simulink model "BLDC_System_Level"  (R2022b)
settings: Solver=FixedStepAuto  StartTime=0.0  StopTime=10.0  RelTol=1e-3
PreLoadFcn:
  | init_params
InitFcn:
  | init_params
undefined symbols (not defined in the file): V_dc
settings Model: Creator=Ahmed Aboeita  LastModifiedBy=Ahmed Aboeita

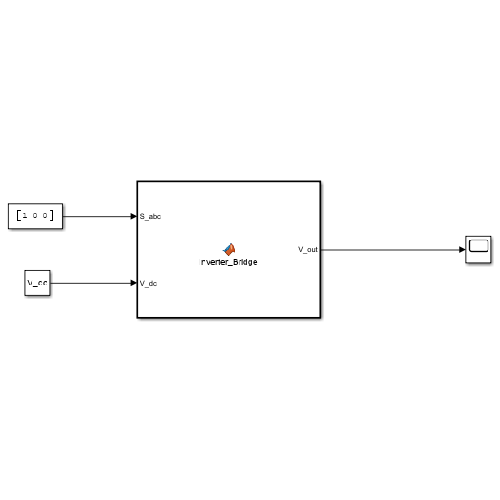
[thumbnail: Simulink's stored preview of the top-level diagram]
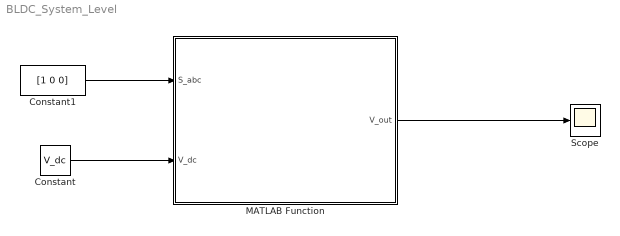
== system BLDC_System_Level ==
  Constant : Constant  Value=V_dc
  Constant1 : Constant  Value=[1 0 0]
  MATLAB Function : MATLAB Function  TreatAsAtomicUnit=on
  Scope : Scope
  wires:
  Constant/1 -> MATLAB Function/2(V_dc)
  Constant1/1 -> MATLAB Function/1(S_abc)
  MATLAB Function/1(V_out) -> Scope/1

== matlab function BLDC_System_Level/MATLAB Function ==
  data: S_abc input; V_out output; V_dc input
function V_out = Inverter_Bridge(S_abc, V_dc)

    % Call the external script in the Functions folder
    V_out = inverter_bridge_logic(S_abc, V_dc);
end
